simulink model "Schimmel_Evan_lab_2_model"  (R2020b)
settings: Solver=VariableStepAuto  StartTime=0.0  StopTime=10.0  RelTol=1e-3
values from neighbouring files (symbols this model uses):
  J = (mp*lp^2)/12+mp*lpcg^2+(1/2)*mw*(dw/2)^2+mw*lwcg^2    (= 7.449551125e-05)    [Schimmel_Evan_lab_2_script.m]
  k = g*(mp*lpcg+mw*lwcg)    (= 0.03094049475)    [Schimmel_Evan_lab_2_script.m]
  omega0 = 0    [Schimmel_Evan_lab_2_script.m]
  theta0 = -Pi/2    [Schimmel_Evan_lab_2_script.m]
settings Model: Creator=schimmer  LastModifiedBy=schimmer

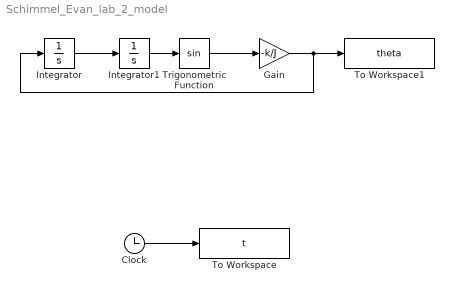
== system Schimmel_Evan_lab_2_model ==
  Clock : Clock
  Gain : Gain  Gain=-k/J
  Integrator : Integrator  InitialCondition=omega0
  Integrator1 : Integrator  InitialCondition=theta0
  To Workspace : ToWorkspace  VariableName=t  SampleTime=-1
  To Workspace1 : ToWorkspace  VariableName=theta  SampleTime=-1
  Trigonometric Function : Trigonometry
  wires:
  Integrator/1 -> Integrator1/1
  Integrator1/1 -> Trigonometric Function/1
  Trigonometric Function/1 -> Gain/1
  Gain/1 -> To Workspace1/1, Integrator/1
  Clock/1 -> To Workspace/1
